simulink model "RemoteMicrogrid"  (R2025a)
settings: Solver=FixedStepAuto  StartTime=0.0  StopTime=8  FixedStep=Ts  MaxStep=1e-3  RelTol=1e-3
PreLoadFcn:
  | RemoteMicrogridInputData
undefined symbols (not defined in the file): BESS, ControlRoom, DiscIntNeverNeededParam, Grid, Load, Machine, Microgrid, MicrogridStatus, PV, relay1, T_on, Ts
libraries: ee_lib x53, fl_lib x39, eeGeneralControl x30, simulink x30, nesl_utility x26, nesl_utility_internal x19, slpidlib x7, eeTransforms x5, eeRmsMeasurement x4, eeTotalHarmonicDistorsion x4, batteryecm_lib x2, simulink_extras x2
(part 2 of 6)

== system RemoteMicrogrid/Diesel Substation, BESS, & Microgrid Controller/Diesel Generator ==
  Bus Element In : Inport  PortName=MGController  Element=Status.loadReference
  AVR and Exciter : Subsystem
  Add : Sum
  Constant : Constant  Value=Machine.LoadReference
  "Governor and Prime Mover " : Subsystem  mask(Governor and Prime Mover){pu_speed_reference=Machine.SpeedReference, droop_percentage=Machine.Droop, pu_load_reference_setpoint=Machine.LoadReference, T_G=Machine.TimeConstandGovernor, T_CH=Machine.TimeConstantPrimeMover, base_torque=Machine.BaseTorque, pu_torque0=Machine.InitialTorque}
      mask prompts: pu_speed_reference "Speed reference, (pu)"; droop_percentage "Percentage droop, (%)"; pu_load_reference_setpoint "Load reference setpoint, (pu)"; T_G "Time constant of governor, (s)"; T_CH "Time constant of main inlet volumes and steam chest, (s)"; base_torque "Base torque, (N*m)"; pu_torque0 "Initial torque, (pu)"
      mask help:
      | Implements a synchronous machine governor and prime mover. The prime mover is a non-reheat steam turbine.
      |
      | The input to the block is a per-unit synchronous machine measurement vector.
      |
      | R and C are mechanical rotational ports.
  Machine Inertia : ee_lib/Electromechanical/Mechanical/Machine Inertia  SRated=Grid.DieselRatedPower V*A  FRated=Grid.Frequency Hz  nPolePairs=1  inertia_option=1  J=Machine.Inertia kg*m^2  H=3.525 s*W/V/A  damper_option=2  D=39.0509 N*m/(rad/s)  pu_D=0.01  initialization_option=2  fMechanical0=60 Hz  fElectrical0=Grid.Frequency Hz
      settings: InternalSimscapePortConfiguration="{\"Bottom\":[],\"Left\":[{\"id\":\"R\",\"label\":\"R\",\"type\":\"foundation.mechanical.rotational.rotational\"}],\"Right\":[],\"Top\":[]}"
  Synchronous Machine Round Rotor : ee_lib/Electromechanical/Synchronous/Synchronous Machine Round Rotor  port_option=ee.enum.threePhasePort.composite  SRated=Grid.DieselRatedPower A*V  VRated=Grid.Voltage V  FRated=Grid.Frequency Hz  nPolePairs=1  param_option=ee.enum.sm.parameterization.standard  fieldCircuitParameterization_option=ee.enum.sm.fieldparameterization.current  baseEfd=92.95 V  baseIfd=1300 A  zero_sequence=ee.enum.park.zerosequence.include  axes_param=ee.enum.rotorangle.daxis  Ladu=1.66  Laqu=1.61  L0=0.15  Ll=0.05  Ra=0.03  Lfd=0.165  Rfd=0.0006  L1d=0.1713  R1d=0.0284  L1q=0.7252  R1q=0.00619  L2q=0.125  R2q=0.02368  Xl=0.05  Xd=1.72  Xq=0.79  X0=0.06  Xdd=0.13  Xqd=0.17  Xddd=0.09  Xqdd=0.12  d_option=ee.enum.circuit.open  Td0d=0.75 s  Tdd=0.03 s  Td0dd=0.03 s  Tddd=0.008 s  q_option=ee.enum.circuit.open  Tq0d=0.6 s  Tqd=0.03 s  Tq0dd=0.02 s  Tqdd=0.008 s  saturation_option=ee.enum.saturation.exclude  saturation_ifd=[0, .48, .76, 1.38, 1.79]  saturation_Vag=[0, .8, 1.08, 1.31, 1.4]  initialization_option=ee.enum.sm.initialization.steadystate  source_type=ee.enum.sm.load_flow_source_type.Swing  Vmag0=Grid.Voltage V  Vang0=0 deg  Pt0=Grid.DieselRatedPower A*V  Qt0=0 A*V  minimum_pu=0.95  phase_search_range=[-inf, inf] deg  gmin=1e-6 S  connection_option=ee.enum.Connection.wye  num_q_dampers=2  rotor_offset=-pi / 2 rad  pu_psid_specify=off  pu_psid_priority=None  pu_psid=0  pu_psid_nominal_specify=off  pu_psid_nominal_value=1  pu_psid_nominal_unit=1  pu_psiq_specify=off  pu_psiq_priority=None  pu_psiq=0  pu_psiq_nominal_specify=off  pu_psiq_nominal_value=1  pu_psiq_nominal_unit=1  pu_psifd_specify=off  pu_psifd_priority=None  pu_psifd=0  pu_psifd_nominal_specify=off  pu_psifd_nominal_value=1  pu_psifd_nominal_unit=1  pu_psi1d_specify=off  pu_psi1d_priority=None  pu_psi1d=0  pu_psi1d_nominal_specify=off  pu_psi1d_nominal_value=1  pu_psi1d_nominal_unit=1  pu_psi1q_specify=off  pu_psi1q_priority=None  pu_psi1q=0  pu_psi1q_nominal_specify=off  pu_psi1q_nominal_value=1  pu_psi1q_nominal_unit=1  pu_psi2q_specify=off  pu_psi2q_priority=None  pu_psi2q=0  pu_psi2q_nominal_specify=off  pu_psi2q_nominal_value=1  pu_psi2q_nominal_unit=1  angular_position_diff_specify=off  angular_position_diff_priority=None  angular_position_diff=180 deg  angular_position_diff_nominal_specify=off  angular_position_diff_nominal_value=1  angular_position_diff_nominal_unit=deg  Tmeas=298.15 K  alpha=3.93e-3 1/K  stator_thermal_mass=100 J/K  rotor_thermal_mass=200 J/K  temperatureA_specify=off  temperatureA_priority=High  temperatureA=25 degC  temperatureA_nominal_specify=off  temperatureA_nominal_value=1  temperatureA_nominal_unit=degC  temperatureB_specify=off  temperatureB_priority=High  temperatureB=25 degC  temperatureB_nominal_specify=off  temperatureB_nominal_value=1  temperatureB_nominal_unit=degC  temperatureC_specify=off  temperatureC_priority=High  temperatureC=25 degC  temperatureC_nominal_specify=off  temperatureC_nominal_value=1  temperatureC_nominal_unit=degC  temperatureR_specify=off  temperatureR_priority=High  temperatureR=25 degC  temperatureR_nominal_specify=off  temperatureR_nominal_value=1  temperatureR_nominal_unit=degC
      settings: InternalSimscapePortConfiguration="{\"Bottom\":[],\"Left\":[{\"id\":\"fd_p\",\"label\":\"fd+\",\"type\":\"foundation.electrical.electrical\"},{\"id\":\"fd_n\",\"label\":\"fd-\",\"type\":\"foundation.electrical.electrical\"},{\"id\":\"R\",\"label\":\"R\",\"type\":\"foundation.mechanical.rotational.rotational\"},{\"id\":\"C\",\"label\":\"C\",\"type\":\"foundation.mechanical.rotational.rotational\"}],\"Right\":[{\"id\":\"pu_output\",\"label\":\"pu\",\"type\":\"output\"},{\"id\":\"N\",\"label\":\"~\",\"type\":\"foundation.electrical.three_phase\"},{\"id\":\"n\",\"label\":\"n\",\"type\":\"foundation.electrical.electrical\"}],\"Top\":[]}"
  ref : PMIOPort  Side=Left
  ~ : PMIOPort  Port=2  Side=Right
  wires:
  Add/1 -> "Governor and Prime Mover "/1(Load)
  Constant/1 -> Add/2
  Bus Element In/1 -> Add/1
  connections:
  AVR and Exciter/LConn1 -- "Governor and Prime Mover "/LConn1 -- Synchronous Machine Round Rotor/RConn1
  Synchronous Machine Round Rotor/LConn3 -- Machine Inertia/LConn1 -- "Governor and Prime Mover "/RConn1
  Synchronous Machine Round Rotor/LConn1 -- AVR and Exciter/RConn1
  AVR and Exciter/RConn2 -- Synchronous Machine Round Rotor/RConn3 -- ref/RConn1 -- Synchronous Machine Round Rotor/LConn2
  Synchronous Machine Round Rotor/LConn4 -- "Governor and Prime Mover "/RConn2
  Synchronous Machine Round Rotor/RConn2 -- ~/RConn1

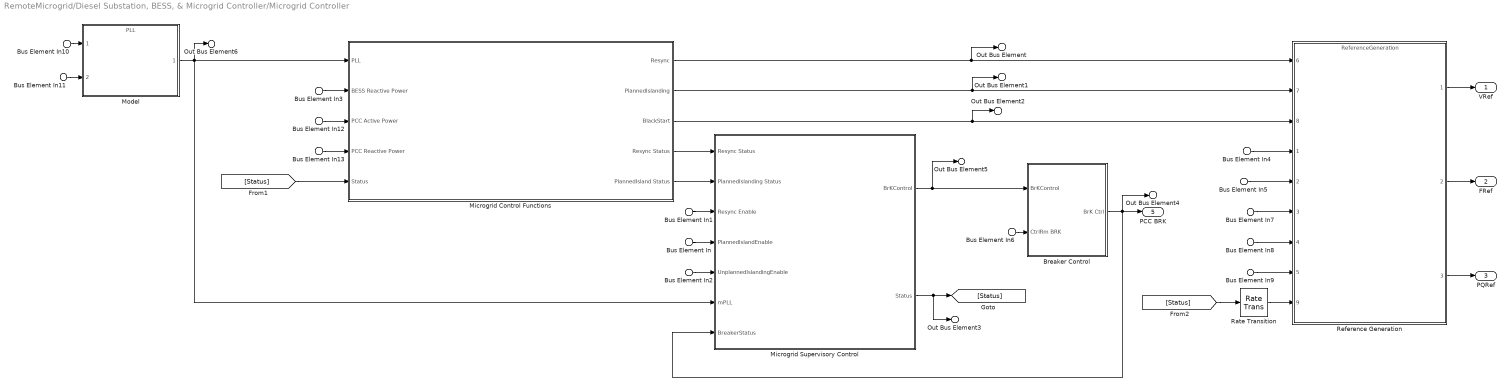
== system RemoteMicrogrid/Diesel Substation, BESS, & Microgrid Controller/Microgrid Controller ==
  Bus Element In3 : Inport  PortName=CtrlRmSubstation  Element=BESSReactivePower
  Bus Element In4 : Inport  PortName=CtrlRmSubstation  Element=Pref
  Bus Element In5 : Inport  PortName=CtrlRmSubstation  Element=Qref
  Bus Element In7 : Inport  PortName=CtrlRmSubstation  Element=Vref
  Bus Element In8 : Inport  PortName=CtrlRmSubstation  Element=Fref
  Bus Element In9 : Inport  PortName=CtrlRmSubstation  Element=PowerCmd
  Bus Element In : Inport  PortName=CtrlRmSubstation  Element=PlannedIslandCmd
  Bus Element In1 : Inport  PortName=CtrlRmSubstation  Element=ResynchCmd
  Bus Element In2 : Inport  PortName=CtrlRmSubstation  Element=UnplannedIslanding
  Bus Element In6 : Inport  PortName=CtrlRmSubstation  Element=BRKcontrol
  Bus Element In10 : Inport  Port=2  PortName=mPCC  Element=Grid.voltage
  Bus Element In11 : Inport  Port=2  PortName=mPCC  Element=PCC.voltage
  Bus Element In12 : Inport  Port=2  PortName=mPCC  Element=PCC.activePower
  Bus Element In13 : Inport  Port=2  PortName=mPCC  Element=PCC.reactivePower
  Breaker Control : Subsystem  mask(Breaker Control){}
      mask help: Control breaker at PCC
  Microgrid Control Functions : Subsystem
  Microgrid Supervisory Control : Subsystem
  Model : ModelReference  ModelNameDialog=PLL.slx  UsingDefaultArgumentValue=0,0,0  SimulationMode=Normal  ModelReferenceVersion=5.0  GridFrequency=gridFrequency  KiPLLController=kpPLL  KpPLLController=kiPLL
  Rate Transition : RateTransition  OutPortSampleTime=1e-3
  Reference Generation : ModelReference  ModelNameDialog=ReferenceGeneration.slx  UsingDefaultArgumentValue=0,0,0,0,0  SimulationMode=Normal  ModelReferenceVersion=5.0  GridFrequency=gridFrequency  pUpperLimit=pUpperLimit  pLowerLimit=pLowerLimit  qUpperLimit=qUpperLimit  qLowerLimit=qLowerLimit
      settings: PortSchema="{\"entries\":[{\"content\":{\"sides\":[{\"content\":{\"connectorIds\":[\"In6\",\"In7\",\"In8\",\"In1\",\"In2\",\"In3\",\"In4\",\"In5\",\"In9\"]},\"type\":\"ConnectorPlacement.EquallySpacedRectSide\",\"uuid\":\"e872b833-49f6-4912-b4b3-51343786db27\"},{\"content\":{\"connectorIds\":[\"Out1\",\"Out2\",\"Out3\"],\"side\":\"RIGHT\"},\"type\":\"ConnectorPlacement.EquallySpacedRectSide\",\"uuid\":\"d01ecec0-b655-4b5d-a34d-324f522879ad\"},{\"content\":{\"side\":\"TOP\"},\"type\":\"ConnectorPlacement.EquallySpacedRectSide\",\"uuid\":\"07b88f4e-1122-4691-94e1-fc20c2cbb47d\"}]},\"type\":\"ConnectorPlacement.EquallySpacedConnector\",\"uuid\":\"8d1da379-bdae-48c1-83d9-0dc3b93882b1\"}],\"packageUris\":[\"http://schema.mathworks.com/mf0/Connector/R2020b\"],\"version\":\"1.0\"}"
  VRef : Outport
  FRef : Outport  Port=2
  PQRef : Outport  Port=3
  Out Bus Element : Outport  Port=4  PortName=MGController  Element=Resync
  Out Bus Element1 : Outport  Port=4  PortName=MGController  Element=PlannedIslanding
  Out Bus Element2 : Outport  Port=4  PortName=MGController  Element=BlackStart
  Out Bus Element3 : Outport  Port=4  PortName=MGController  Element=Status
  Out Bus Element4 : Outport  Port=4  PortName=MGController  Element=BRK Status
  Out Bus Element6 : Outport  Port=4  PortName=MGController  Element=mPLL
  Out Bus Element5 : Outport  Port=4  PortName=MGController  Element=BrKControl
  PCC BRK : Outport  Port=5
  wires:
  Bus Element In7/1 -> Reference Generation/3
  Reference Generation/2 -> FRef/1
  Bus Element In8/1 -> Reference Generation/4
  Bus Element In3/1 -> Microgrid Control Functions/2(BESS Reactive Power)
  Reference Generation/1 -> VRef/1
  Reference Generation/3 -> PQRef/1
  Bus Element In12/1 -> Microgrid Control Functions/3(PCC Active Power)
  Bus Element In4/1 -> Reference Generation/1
  Bus Element In13/1 -> Microgrid Control Functions/4(PCC Reactive Power)
  Bus Element In10/1 -> Model/1
  Bus Element In5/1 -> Reference Generation/2
  Bus Element In2/1 -> Microgrid Supervisory Control/5(UnplannedIslandingEnable)
  Bus Element In/1 -> Microgrid Supervisory Control/4(PlannedIslandEnable)
  Bus Element In11/1 -> Model/2
  Bus Element In9/1 -> Reference Generation/5
  Bus Element In1/1 -> Microgrid Supervisory Control/3(Resync Enable)
  Microgrid Supervisory Control/1(BrKControl) -> Out Bus Element5/1, Breaker Control/1(BrKControl)
  Bus Element In6/1 -> Breaker Control/2(CtrlRm BRK)
  Model/1 -> Out Bus Element6/1, Microgrid Supervisory Control/6(mPLL), Microgrid Control Functions/1(PLL)
  Microgrid Control Functions/2(PlannedIslanding) -> Out Bus Element1/1, Reference Generation/7
  Microgrid Control Functions/1(Resync) -> Out Bus Element/1, Reference Generation/6
  Microgrid Control Functions/4(Resync Status) -> Microgrid Supervisory Control/1(Resync Status)
  Microgrid Control Functions/5(PlannedIsland Status) -> Microgrid Supervisory Control/2(PlannedIslanding Status)
  Breaker Control/1(BrK Ctrl) -> Microgrid Supervisory Control/7(BreakerStatus), PCC BRK/1, Out Bus Element4/1
  Microgrid Control Functions/3(BlackStart) -> Out Bus Element2/1, Reference Generation/8
  Microgrid Supervisory Control/2(Status) -> Out Bus Element3/1, [Status]
  [Status] -> Microgrid Control Functions/5(Status)
  [Status] -> Rate Transition/1
  Rate Transition/1 -> Reference Generation/9

== system RemoteMicrogrid/Diesel Substation, BESS, & Microgrid Controller/PCC Measurements and PCC Breaker ==
  Breaker : Inport
  Bus Creator : BusCreator  Inputs=2
  Circuit Breaker : Subsystem
  Diesel Genset Current Measurement : Subsystem
  Diesel Genset Power Measurement : Subsystem
  ~ : PMIOPort  Side=Left
  "~ " : PMIOPort  Port=2  Side=Right
  " mPCC" : Outport
  wires:
  Bus Creator/1 -> " mPCC"/1  "mPCC"
  Diesel Genset Power Measurement/1(PCC) -> Bus Creator/2  "PCC"
  Diesel Genset Current Measurement/1(Grid) -> Bus Creator/1  "Grid"
  Breaker/1 -> Circuit Breaker/1(BRK)
  connections:
  Circuit Breaker/LConn1 -- Diesel Genset Current Measurement/RConn1
  Diesel Genset Power Measurement/RConn1 -- "~ "/RConn1
  ~/RConn1 -- Diesel Genset Current Measurement/LConn1
  Circuit Breaker/RConn1 -- Diesel Genset Power Measurement/LConn1

== system RemoteMicrogrid/Diesel Substation, BESS, & Microgrid Controller/Transformer and Disconnectors ==
  Connectors : ee_lib/Passive/RLC Assemblies/RLC (Three-Phase)  port_option=ee.enum.threePhasePort.composite  component_structure=ee.enum.rlc.structure.R  R=Grid.ConnectorResistance Ohm  L=0.01 H  C=1e-6 F  R_parasitic=1e-6 Ohm  G_parasitic=1e-6 1/Ohm  IL_specify=on  IL_priority=High  IL=[0, 0, 0] A  IL_nominal_specify=off  IL_nominal_value=1  IL_nominal_unit=A  VC_specify=off  VC_priority=High  VC=[0, 0, 0] V  VC_nominal_specify=off  VC_nominal_value=1  VC_nominal_unit=V
      settings: InternalSimscapePortConfiguration="{\"Bottom\":[],\"Left\":[{\"id\":\"N1\",\"label\":\"~1\",\"type\":\"foundation.electrical.three_phase\"}],\"Right\":[{\"id\":\"N2\",\"label\":\"~2\",\"type\":\"foundation.electrical.three_phase\"}],\"Top\":[]}"
  Electrical Reference5 : fl_lib/Electrical/Electrical Elements/Electrical Reference
  Fault (Three-Phase) : ee_lib/Utilities/Fault (Three-Phase)  fault_type_option=1  R_pn_fault=50 Ohm  R_ng_fault=1e-3 Ohm  exposemeasurement=ee.enum.exposemeasurement.hidden  enable_external_fault=ee.enum.external_fault.hidden  fault_threshold=0.5  fault_condition=1  fault_resettable=1  enable_temporal_fault=1  fault_start_time=ControlRoom.unplannedIslanding s  fault_duration=0.3 s  G_parasitic=1e-6 1/Ohm
      settings: InternalSimscapePortConfiguration="{\"Bottom\":[],\"Left\":[{\"id\":\"N\",\"label\":\"~\",\"type\":\"foundation.electrical.three_phase\"}],\"Right\":[],\"Top\":[]}"
  Switchable 20 kW 4160 Vrms 60 Hz1 : ee_lib/Passive/RLC Assemblies/Wye-Connected Load  port_option=ee.enum.threePhasePort.composite  parameterization=ee.enum.rlc.parameterization.ratedpower  component_structure=ee.enum.rlc.structure.C  component_structure_PQ=ee.enum.rlc.structure.R  R=1 Ohm  L=0.001 H  C=1e-6 F  VRated=Microgrid.Voltage V  FRated=Grid.Frequency Hz  P=20000 W  Qpos=0 A*V  Qneg=-30000 A*V  R_parasitic=1e-6 Ohm  G_parasitic=1e-6 1/Ohm  R_parasitic_PQ=1e-6 Ohm  G_parasitic_PQ=1e-6 1/Ohm  Vmag0=Microgrid.Voltage V  Vang0=0 deg  Freq0=Microgrid.Frequency Hz  IL_specify=on  IL_priority=High  IL=[ 0 0 0 ] A  IL_nominal_specify=off  IL_nominal_value=1  IL_nominal_unit=A  VC_specify=on  VC_priority=High  VC=[ 0 0 0 ] V  VC_nominal_specify=off  VC_nominal_value=1  VC_nominal_unit=V
  Two-Winding Transformer (Three-Phase)1 : ee_lib/Passive/Transformers/Two-Winding Transformer (Three-Phase)  SRated=Grid.TransformerRating A*V  FRated=Grid.Frequency Hz  Winding1Connection=ee.enum.windingconnection.Y  VRated1=Grid.TransformerPrimaryVoltage V  Winding2Connection=ee.enum.windingconnection.Y  VRated2=Grid.TransformerSecondaryVoltage V  CoreType=ee.enum.coretype.threelimb  pu_Rw1=Grid.Primaryresistance  pu_Rw2=Grid.Secondaryresistance  leakage_reactance_option=ee.enum.transformer_leakage.include  pu_Xl1=Grid.Primaryreactance  pu_Xl2=Grid.Secondaryreactance  magnetizing_resistance_option=ee.enum.transformer_magnetizingResistance.include  pu_Rm=500  magnetizing_reactance_option=ee.enum.transformer_magnetizingReactance.include  saturation_option=ee.enum.transformer_saturation.exclude  pu_Xm=500  current_data=[0, .002, 1, 2]  magnetic_flux_data=[0, 1.2, 1.5, 1.51]  pu_X0=0.5  i1_specify=on  i1_priority=None  i1=[0, 0, 0] A  i1_nominal_specify=off  i1_nominal_value=1  i1_nominal_unit=A  i2_specify=on  i2_priority=None  i2=[0, 0, 0] A  i2_nominal_specify=off  i2_nominal_value=1  i2_nominal_unit=A  phi_specify=off  phi_priority=None  phi=[0, 0, 0]  phi_nominal_specify=off  phi_nominal_value=1  phi_nominal_unit=1  power_dissipated_specify=off  power_dissipated_priority=None  power_dissipated=0 W  power_dissipated_nominal_specify=off  power_dissipated_nominal_value=1  power_dissipated_nominal_unit=W
      settings: InternalSimscapePortConfiguration="{\"Bottom\":[],\"Left\":[{\"id\":\"N1\",\"label\":\"~1\",\"type\":\"foundation.electrical.three_phase\"}],\"Right\":[{\"id\":\"N2\",\"label\":\"~2\",\"type\":\"foundation.electrical.three_phase\"}],\"Top\":[]}"
  ~ : PMIOPort  Side=Left
  "~ " : PMIOPort  Port=2  Side=Right
  connections:
  Connectors/LConn1 -- Two-Winding Transformer (Three-Phase)1/RConn1
  Switchable 20 kW 4160 Vrms 60 Hz1/LConn1 -- "~ "/RConn1 -- Fault (Three-Phase)/LConn1 -- Connectors/RConn1
  Switchable 20 kW 4160 Vrms 60 Hz1/RConn1 -- Electrical Reference5/LConn1
  ~/RConn1 -- Two-Winding Transformer (Three-Phase)1/LConn1

== system RemoteMicrogrid/Feeder 2B & NO Switch/Circuit Breaker ==
  BRK : Inport
  Data Type Conversion : DataTypeConversion  OutDataTypeStr=double  SaturateOnIntegerOverflow=off  RndMeth=Floor
  Open Resistance : Gain  Gain=1e5
  Phase Splitter : ee_lib/Connectors & References/Phase Splitter
  Phase Splitter1 : ee_lib/Connectors & References/Phase Splitter
  Simulink-PS Converter : nesl_utility/Simulink-PS Converter  PhysicalDomain=network_engine_domain  SubClassName=ps_input  LeftPortType=input  RightPortType=output  PseudoPeriodic=off  Frequencies=[]  NoiseDistribution=none  NoiseParameters=[]  Unit=1  AffineConversion=off  FilteringAndDerivatives=provide  SimscapeFilterOrder=1  InputFilterTimeConstant=0.001  UdotUserProvided=0
  Variable Resistor : fl_lib/Electrical/Electrical Elements/Variable Resistor  Rmin=1e-3 Ohm  thermalEnable=false  thermal_mass=1 J/K  i_specify=off  i_priority=None  i=0 A  i_nominal_specify=off  i_nominal_value=1  i_nominal_unit=A  v_specify=off  v_priority=None  v=0 V  v_nominal_specify=off  v_nominal_value=1  v_nominal_unit=V  T_specify=off  T_priority=None  T=300 K  T_nominal_specify=off  T_nominal_value=1  T_nominal_unit=K
  Variable Resistor1 : fl_lib/Electrical/Electrical Elements/Variable Resistor  Rmin=1e-3 Ohm  thermalEnable=false  thermal_mass=1 J/K  i_specify=off  i_priority=None  i=0 A  i_nominal_specify=off  i_nominal_value=1  i_nominal_unit=A  v_specify=off  v_priority=None  v=0 V  v_nominal_specify=off  v_nominal_value=1  v_nominal_unit=V  T_specify=off  T_priority=None  T=300 K  T_nominal_specify=off  T_nominal_value=1  T_nominal_unit=K
  Variable Resistor2 : fl_lib/Electrical/Electrical Elements/Variable Resistor  Rmin=1e-3 Ohm  thermalEnable=false  thermal_mass=1 J/K  i_specify=off  i_priority=None  i=0 A  i_nominal_specify=off  i_nominal_value=1  i_nominal_unit=A  v_specify=off  v_priority=None  v=0 V  v_nominal_specify=off  v_nominal_value=1  v_nominal_unit=V  T_specify=off  T_priority=None  T=300 K  T_nominal_specify=off  T_nominal_value=1  T_nominal_unit=K
  In : PMIOPort  Side=Left
  ~ : PMIOPort  Port=2  Side=Right
  wires:
  Data Type Conversion/1 -> Open Resistance/1
  BRK/1 -> Data Type Conversion/1
  Open Resistance/1 -> Simulink-PS Converter/1
  connections:
  Phase Splitter1/RConn2 -- Variable Resistor1/RConn1
  Variable Resistor1/LConn2 -- Phase Splitter/RConn2
  Phase Splitter1/RConn3 -- Variable Resistor2/RConn1
  Phase Splitter/RConn1 -- Variable Resistor/LConn2
  Variable Resistor2/LConn2 -- Phase Splitter/RConn3
  Phase Splitter1/RConn1 -- Variable Resistor/RConn1
  Phase Splitter1/LConn1 -- ~/RConn1
  Variable Resistor/LConn1 -- Simulink-PS Converter/RConn1 -- Variable Resistor2/LConn1 -- Variable Resistor1/LConn1
  Phase Splitter/LConn1 -- In/RConn1

== system RemoteMicrogrid/Feeder 2B & NO Switch/Circuit Breaker1 ==
  BRK : Inport
  Data Type Conversion : DataTypeConversion  OutDataTypeStr=double  SaturateOnIntegerOverflow=off  RndMeth=Floor
  Open Resistance : Gain  Gain=1e5
  Phase Splitter : ee_lib/Connectors & References/Phase Splitter
  Phase Splitter1 : ee_lib/Connectors & References/Phase Splitter
  Simulink-PS Converter : nesl_utility/Simulink-PS Converter  PhysicalDomain=network_engine_domain  SubClassName=ps_input  LeftPortType=input  RightPortType=output  PseudoPeriodic=off  Frequencies=[]  NoiseDistribution=none  NoiseParameters=[]  Unit=1  AffineConversion=off  FilteringAndDerivatives=provide  SimscapeFilterOrder=1  InputFilterTimeConstant=0.001  UdotUserProvided=0
  Variable Resistor : fl_lib/Electrical/Electrical Elements/Variable Resistor  Rmin=1e-3 Ohm  thermalEnable=false  thermal_mass=1 J/K  i_specify=off  i_priority=None  i=0 A  i_nominal_specify=off  i_nominal_value=1  i_nominal_unit=A  v_specify=off  v_priority=None  v=0 V  v_nominal_specify=off  v_nominal_value=1  v_nominal_unit=V  T_specify=off  T_priority=None  T=300 K  T_nominal_specify=off  T_nominal_value=1  T_nominal_unit=K
  Variable Resistor1 : fl_lib/Electrical/Electrical Elements/Variable Resistor  Rmin=1e-3 Ohm  thermalEnable=false  thermal_mass=1 J/K  i_specify=off  i_priority=None  i=0 A  i_nominal_specify=off  i_nominal_value=1  i_nominal_unit=A  v_specify=off  v_priority=None  v=0 V  v_nominal_specify=off  v_nominal_value=1  v_nominal_unit=V  T_specify=off  T_priority=None  T=300 K  T_nominal_specify=off  T_nominal_value=1  T_nominal_unit=K
  Variable Resistor2 : fl_lib/Electrical/Electrical Elements/Variable Resistor  Rmin=1e-3 Ohm  thermalEnable=false  thermal_mass=1 J/K  i_specify=off  i_priority=None  i=0 A  i_nominal_specify=off  i_nominal_value=1  i_nominal_unit=A  v_specify=off  v_priority=None  v=0 V  v_nominal_specify=off  v_nominal_value=1  v_nominal_unit=V  T_specify=off  T_priority=None  T=300 K  T_nominal_specify=off  T_nominal_value=1  T_nominal_unit=K
  In : PMIOPort  Side=Left
  ~ : PMIOPort  Port=2  Side=Right
  wires:
  Data Type Conversion/1 -> Open Resistance/1
  BRK/1 -> Data Type Conversion/1
  Open Resistance/1 -> Simulink-PS Converter/1
  connections:
  Phase Splitter1/RConn2 -- Variable Resistor1/RConn1
  Variable Resistor1/LConn2 -- Phase Splitter/RConn2
  Phase Splitter1/RConn3 -- Variable Resistor2/RConn1
  Phase Splitter/RConn1 -- Variable Resistor/LConn2
  Variable Resistor2/LConn2 -- Phase Splitter/RConn3
  Phase Splitter1/RConn1 -- Variable Resistor/RConn1
  Phase Splitter1/LConn1 -- ~/RConn1
  Variable Resistor/LConn1 -- Simulink-PS Converter/RConn1 -- Variable Resistor2/LConn1 -- Variable Resistor1/LConn1
  Phase Splitter/LConn1 -- In/RConn1

== system RemoteMicrogrid/Feeder 2B & NO Switch/Subsystem ==
  ControlRoom : Inport
  Data Type Conversion1 : DataTypeConversion  SaturateOnIntegerOverflow=off  RndMeth=Floor
  Delay : Delay  DelayLength=6  SampleTime=0.15
  Logical Operator : Logic  Operator=NOT  AllPortsSameDT=off  OutDataTypeStr=boolean
  Output : Outport
  Output1 : Outport  Port=2
  wires:
  ControlRoom/1 -> Logical Operator/1, Delay/1
  Data Type Conversion1/1 -> Output1/1
  Delay/1 -> Data Type Conversion1/1
  Logical Operator/1 -> Output/1

== system RemoteMicrogrid/LV Load /Circuit Breaker ==
  BRK : Inport
  Data Type Conversion : DataTypeConversion  OutDataTypeStr=double  SaturateOnIntegerOverflow=off  RndMeth=Floor
  Gain : Gain  Gain=9.9e4
  Phase Splitter : ee_lib/Connectors & References/Phase Splitter
  Phase Splitter1 : ee_lib/Connectors & References/Phase Splitter
  Simulink-PS Converter : nesl_utility/Simulink-PS Converter  PhysicalDomain=network_engine_domain  SubClassName=ps_input  LeftPortType=input  RightPortType=output  PseudoPeriodic=off  Frequencies=[]  NoiseDistribution=none  NoiseParameters=[]  Unit=1  AffineConversion=off  FilteringAndDerivatives=provide  SimscapeFilterOrder=1  InputFilterTimeConstant=0.001  UdotUserProvided=0
  Variable Resistor : fl_lib/Electrical/Electrical Elements/Variable Resistor  Rmin=1e-3 Ohm  thermalEnable=false  thermal_mass=1 J/K  i_specify=off  i_priority=None  i=0 A  i_nominal_specify=off  i_nominal_value=1  i_nominal_unit=A  v_specify=off  v_priority=None  v=0 V  v_nominal_specify=off  v_nominal_value=1  v_nominal_unit=V  T_specify=off  T_priority=None  T=300 K  T_nominal_specify=off  T_nominal_value=1  T_nominal_unit=K
  Variable Resistor1 : fl_lib/Electrical/Electrical Elements/Variable Resistor  Rmin=1e-3 Ohm  thermalEnable=false  thermal_mass=1 J/K  i_specify=off  i_priority=None  i=0 A  i_nominal_specify=off  i_nominal_value=1  i_nominal_unit=A  v_specify=off  v_priority=None  v=0 V  v_nominal_specify=off  v_nominal_value=1  v_nominal_unit=V  T_specify=off  T_priority=None  T=300 K  T_nominal_specify=off  T_nominal_value=1  T_nominal_unit=K
  Variable Resistor2 : fl_lib/Electrical/Electrical Elements/Variable Resistor  Rmin=1e-3 Ohm  thermalEnable=false  thermal_mass=1 J/K  i_specify=off  i_priority=None  i=0 A  i_nominal_specify=off  i_nominal_value=1  i_nominal_unit=A  v_specify=off  v_priority=None  v=0 V  v_nominal_specify=off  v_nominal_value=1  v_nominal_unit=V  T_specify=off  T_priority=None  T=300 K  T_nominal_specify=off  T_nominal_value=1  T_nominal_unit=K
  In : PMIOPort  Side=Left
  ~ : PMIOPort  Port=2  Side=Right
  wires:
  Data Type Conversion/1 -> Gain/1
  BRK/1 -> Data Type Conversion/1
  Gain/1 -> Simulink-PS Converter/1
  connections:
  Phase Splitter1/RConn2 -- Variable Resistor1/RConn1
  Variable Resistor1/LConn2 -- Phase Splitter/RConn2
  Phase Splitter1/RConn3 -- Variable Resistor2/RConn1
  Phase Splitter/RConn1 -- Variable Resistor/LConn2
  Variable Resistor2/LConn2 -- Phase Splitter/RConn3
  Phase Splitter1/RConn1 -- Variable Resistor/RConn1
  Phase Splitter1/LConn1 -- ~/RConn1
  Variable Resistor/LConn1 -- Simulink-PS Converter/RConn1 -- Variable Resistor2/LConn1 -- Variable Resistor1/LConn1
  Phase Splitter/LConn1 -- In/RConn1

== system RemoteMicrogrid/LV Load /Circuit Breaker 1 ==
  BRK : Inport
  Data Type Conversion : DataTypeConversion  OutDataTypeStr=double  SaturateOnIntegerOverflow=off  RndMeth=Floor
  Gain : Gain  Gain=9.9e4
  Phase Splitter : ee_lib/Connectors & References/Phase Splitter
  Phase Splitter1 : ee_lib/Connectors & References/Phase Splitter
  Simulink-PS Converter : nesl_utility/Simulink-PS Converter  PhysicalDomain=network_engine_domain  SubClassName=ps_input  LeftPortType=input  RightPortType=output  PseudoPeriodic=off  Frequencies=[]  NoiseDistribution=none  NoiseParameters=[]  Unit=1  AffineConversion=off  FilteringAndDerivatives=provide  SimscapeFilterOrder=1  InputFilterTimeConstant=0.001  UdotUserProvided=0
  Variable Resistor : fl_lib/Electrical/Electrical Elements/Variable Resistor  Rmin=1e-3 Ohm  thermalEnable=false  thermal_mass=1 J/K  i_specify=off  i_priority=None  i=0 A  i_nominal_specify=off  i_nominal_value=1  i_nominal_unit=A  v_specify=off  v_priority=None  v=0 V  v_nominal_specify=off  v_nominal_value=1  v_nominal_unit=V  T_specify=off  T_priority=None  T=300 K  T_nominal_specify=off  T_nominal_value=1  T_nominal_unit=K
  Variable Resistor1 : fl_lib/Electrical/Electrical Elements/Variable Resistor  Rmin=1e-3 Ohm  thermalEnable=false  thermal_mass=1 J/K  i_specify=off  i_priority=None  i=0 A  i_nominal_specify=off  i_nominal_value=1  i_nominal_unit=A  v_specify=off  v_priority=None  v=0 V  v_nominal_specify=off  v_nominal_value=1  v_nominal_unit=V  T_specify=off  T_priority=None  T=300 K  T_nominal_specify=off  T_nominal_value=1  T_nominal_unit=K
  Variable Resistor2 : fl_lib/Electrical/Electrical Elements/Variable Resistor  Rmin=1e-3 Ohm  thermalEnable=false  thermal_mass=1 J/K  i_specify=off  i_priority=None  i=0 A  i_nominal_specify=off  i_nominal_value=1  i_nominal_unit=A  v_specify=off  v_priority=None  v=0 V  v_nominal_specify=off  v_nominal_value=1  v_nominal_unit=V  T_specify=off  T_priority=None  T=300 K  T_nominal_specify=off  T_nominal_value=1  T_nominal_unit=K
  In : PMIOPort  Side=Left
  ~ : PMIOPort  Port=2  Side=Right
  wires:
  Data Type Conversion/1 -> Gain/1
  BRK/1 -> Data Type Conversion/1
  Gain/1 -> Simulink-PS Converter/1
  connections:
  Phase Splitter1/RConn2 -- Variable Resistor1/RConn1
  Variable Resistor1/LConn2 -- Phase Splitter/RConn2
  Phase Splitter1/RConn3 -- Variable Resistor2/RConn1
  Phase Splitter/RConn1 -- Variable Resistor/LConn2
  Variable Resistor2/LConn2 -- Phase Splitter/RConn3
  Phase Splitter1/RConn1 -- Variable Resistor/RConn1
  Phase Splitter1/LConn1 -- ~/RConn1
  Variable Resistor/LConn1 -- Simulink-PS Converter/RConn1 -- Variable Resistor2/LConn1 -- Variable Resistor1/LConn1
  Phase Splitter/LConn1 -- In/RConn1

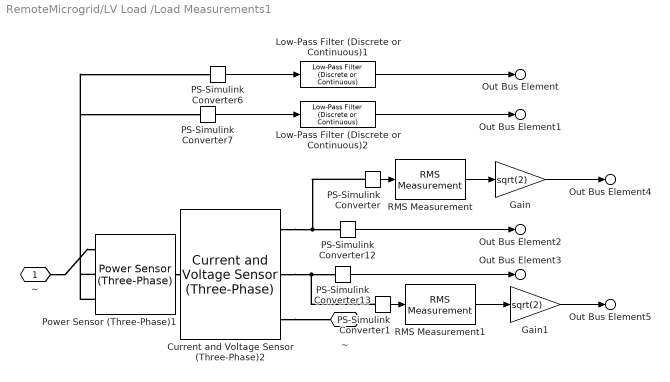
== system RemoteMicrogrid/LV Load /Load Measurements1 ==
  Current and Voltage Sensor (Three-Phase)2 : ee_lib/Sensors & Transducers/Current and Voltage Sensor (Three-Phase)  vMeasurementType=ee.enum.vmeasurement.ll  outputUnit=ee.enum.unit.pu  SRated=150e3 A*V  VRated=Microgrid.LVVoltage V  I_specify=off  I_priority=None  I=[0, 0, 0] A  I_nominal_specify=off  I_nominal_value=1  I_nominal_unit=A  V_specify=off  V_priority=None  V=[0, 0, 0] V  V_nominal_specify=off  V_nominal_value=1  V_nominal_unit=V
      settings: InternalSimscapePortConfiguration="{\"Bottom\":[],\"Left\":[{\"id\":\"N1\",\"label\":\"~1\",\"type\":\"foundation.electrical.three_phase\"}],\"Right\":[{\"id\":\"V_output\",\"label\":\"V\",\"type\":\"output\"},{\"id\":\"I_output\",\"label\":\"I\",\"type\":\"output\"},{\"id\":\"N2\",\"label\":\"~2\",\"type\":\"foundation.electrical.three_phase\"}],\"Top\":[]}"
  Gain : Gain  Gain=sqrt(2)
  Gain1 : Gain  Gain=sqrt(2)
  Low-Pass Filter (Discrete or Continuous)1 : eeGeneralControl/Low-Pass Filter (Discrete or Continuous)  K=1  T=0.02  B=inf  A=-inf  init_option=Inherited from block input  x0=0  Ts=Ts
  Low-Pass Filter (Discrete or Continuous)2 : eeGeneralControl/Low-Pass Filter (Discrete or Continuous)  K=1  T=0.02  B=inf  A=-inf  init_option=Inherited from block input  x0=0  Ts=Ts
  PS-Simulink Converter : nesl_utility/PS-Simulink Converter  PhysicalDomain=network_engine_domain  SubClassName=ps_output  LeftPortType=input  RightPortType=output  PseudoPeriodic=off  Frequencies=[]  VectorFormat=inherit  Unit=inherit  AffineConversion=off
  PS-Simulink Converter1 : nesl_utility/PS-Simulink Converter  PhysicalDomain=network_engine_domain  SubClassName=ps_output  LeftPortType=input  RightPortType=output  PseudoPeriodic=off  Frequencies=[]  VectorFormat=inherit  Unit=inherit  AffineConversion=off
  PS-Simulink Converter12 : nesl_utility_internal/PS-Simulink Converter  PhysicalDomain=network_engine_domain  SubClassName=ps_output  LeftPortType=input  RightPortType=output  PseudoPeriodic=off  Frequencies=[]  VectorFormat=1-D array  Unit=V  AffineConversion=off
  PS-Simulink Converter13 : nesl_utility_internal/PS-Simulink Converter  PhysicalDomain=network_engine_domain  SubClassName=ps_output  LeftPortType=input  RightPortType=output  PseudoPeriodic=off  Frequencies=[]  VectorFormat=1-D array  Unit=A  AffineConversion=off
  PS-Simulink Converter6 : nesl_utility_internal/PS-Simulink Converter  PhysicalDomain=network_engine_domain  SubClassName=ps_output  LeftPortType=input  RightPortType=output  PseudoPeriodic=off  Frequencies=[]  VectorFormat=1-D array  Unit=kW  AffineConversion=off
  PS-Simulink Converter7 : nesl_utility_internal/PS-Simulink Converter  PhysicalDomain=network_engine_domain  SubClassName=ps_output  LeftPortType=input  RightPortType=output  PseudoPeriodic=off  Frequencies=[]  VectorFormat=1-D array  Unit=kV*A  AffineConversion=off
  Power Sensor (Three-Phase)1 : ee_lib/Sensors & Transducers/Power Sensor (Three-Phase)  load_type=ee.enum.passive.type_balanced.balanced  f0=60 Hz  config=ee.enum.with_neutral.no  rho=1
      settings: InternalSimscapePortConfiguration="{\"Bottom\":[],\"Left\":[{\"id\":\"N1\",\"label\":\"~1\",\"type\":\"foundation.electrical.three_phase\"}],\"Right\":[{\"id\":\"N2\",\"label\":\"~2\",\"type\":\"foundation.electrical.three_phase\"}],\"Top\":[{\"id\":\"Pm\",\"label\":\"P\",\"type\":\"output\"},{\"id\":\"Qm\",\"label\":\"Q\",\"type\":\"output\"}]}"
  RMS Measurement : eeRmsMeasurement/RMS Measurement  LabelModeActiveChoice=Total  F=Grid.Frequency  SpecifyHarmonics=off  K=[0 1 2]  Ts=Ts
      settings: LibrarySourceBlock=|
      | ee_sl_lib/Measurements/RMS
      | Measurement
  RMS Measurement1 : eeRmsMeasurement/RMS Measurement  LabelModeActiveChoice=Total  F=Grid.Frequency  SpecifyHarmonics=off  K=[0 1 2]  Ts=Ts
      settings: LibrarySourceBlock=|
      | ee_sl_lib/Measurements/RMS
      | Measurement
  "~ " : PMIOPort  Side=Left
  " ~ " : PMIOPort  Port=2  Side=Right
  Out Bus Element : Outport  PortName=mLoadF2  Element=active powerF2
  Out Bus Element1 : Outport  PortName=mLoadF2  Element=reactive powerF2
  Out Bus Element2 : Outport  PortName=mLoadF2  Element=voltageF2
  Out Bus Element3 : Outport  PortName=mLoadF2  Element=currentF2
  Out Bus Element4 : Outport  PortName=mLoadF2  Element=voltageRMSF2
  Out Bus Element5 : Outport  PortName=mLoadF2  Element=currentRMSF2
  wires:
  Low-Pass Filter (Discrete or Continuous)2/1 -> Out Bus Element1/1
  Low-Pass Filter (Discrete or Continuous)1/1 -> Out Bus Element/1
  PS-Simulink Converter6/1 -> Low-Pass Filter (Discrete or Continuous)1/1
  PS-Simulink Converter7/1 -> Low-Pass Filter (Discrete or Continuous)2/1
  PS-Simulink Converter13/1 -> Out Bus Element3/1
  PS-Simulink Converter12/1 -> Out Bus Element2/1
  PS-Simulink Converter/1 -> RMS Measurement/1
  RMS Measurement/1 -> Gain/1
  RMS Measurement1/1 -> Gain1/1
  PS-Simulink Converter1/1 -> RMS Measurement1/1
  Gain/1 -> Out Bus Element4/1
  Gain1/1 -> Out Bus Element5/1
  connections:
  Power Sensor (Three-Phase)1/RConn1 -- Current and Voltage Sensor (Three-Phase)2/LConn1
  Current and Voltage Sensor (Three-Phase)2/RConn1 -- PS-Simulink Converter/LConn1 -- PS-Simulink Converter12/LConn1
  Current and Voltage Sensor (Three-Phase)2/RConn2 -- PS-Simulink Converter1/LConn1 -- PS-Simulink Converter13/LConn1
  "~ "/RConn1 -- Power Sensor (Three-Phase)1/LConn1
  Current and Voltage Sensor (Three-Phase)2/RConn3 -- " ~ "/RConn1
  Power Sensor (Three-Phase)1/LConn2 -- PS-Simulink Converter6/LConn1
  Power Sensor (Three-Phase)1/LConn3 -- PS-Simulink Converter7/LConn1

== system RemoteMicrogrid/MV Load/Circuit Breaker ==
  BRK : Inport
  Data Type Conversion : DataTypeConversion  OutDataTypeStr=double  SaturateOnIntegerOverflow=off  RndMeth=Floor
  Open Resistance : Gain  Gain=1e5
  Phase Splitter : ee_lib/Connectors & References/Phase Splitter
  Phase Splitter1 : ee_lib/Connectors & References/Phase Splitter
  Simulink-PS Converter : nesl_utility/Simulink-PS Converter  PhysicalDomain=network_engine_domain  SubClassName=ps_input  LeftPortType=input  RightPortType=output  PseudoPeriodic=off  Frequencies=[]  NoiseDistribution=none  NoiseParameters=[]  Unit=1  AffineConversion=off  FilteringAndDerivatives=provide  SimscapeFilterOrder=1  InputFilterTimeConstant=0.001  UdotUserProvided=0
  Variable Resistor : fl_lib/Electrical/Electrical Elements/Variable Resistor  Rmin=1e-3 Ohm  thermalEnable=false  thermal_mass=1 J/K  i_specify=off  i_priority=None  i=0 A  i_nominal_specify=off  i_nominal_value=1  i_nominal_unit=A  v_specify=off  v_priority=None  v=0 V  v_nominal_specify=off  v_nominal_value=1  v_nominal_unit=V  T_specify=off  T_priority=None  T=300 K  T_nominal_specify=off  T_nominal_value=1  T_nominal_unit=K
  Variable Resistor1 : fl_lib/Electrical/Electrical Elements/Variable Resistor  Rmin=1e-3 Ohm  thermalEnable=false  thermal_mass=1 J/K  i_specify=off  i_priority=None  i=0 A  i_nominal_specify=off  i_nominal_value=1  i_nominal_unit=A  v_specify=off  v_priority=None  v=0 V  v_nominal_specify=off  v_nominal_value=1  v_nominal_unit=V  T_specify=off  T_priority=None  T=300 K  T_nominal_specify=off  T_nominal_value=1  T_nominal_unit=K
  Variable Resistor2 : fl_lib/Electrical/Electrical Elements/Variable Resistor  Rmin=1e-3 Ohm  thermalEnable=false  thermal_mass=1 J/K  i_specify=off  i_priority=None  i=0 A  i_nominal_specify=off  i_nominal_value=1  i_nominal_unit=A  v_specify=off  v_priority=None  v=0 V  v_nominal_specify=off  v_nominal_value=1  v_nominal_unit=V  T_specify=off  T_priority=None  T=300 K  T_nominal_specify=off  T_nominal_value=1  T_nominal_unit=K
  In : PMIOPort  Side=Left
  ~ : PMIOPort  Port=2  Side=Right
  wires:
  Data Type Conversion/1 -> Open Resistance/1
  BRK/1 -> Data Type Conversion/1
  Open Resistance/1 -> Simulink-PS Converter/1
  connections:
  Phase Splitter1/RConn2 -- Variable Resistor1/RConn1
  Variable Resistor1/LConn2 -- Phase Splitter/RConn2
  Phase Splitter1/RConn3 -- Variable Resistor2/RConn1
  Phase Splitter/RConn1 -- Variable Resistor/LConn2
  Variable Resistor2/LConn2 -- Phase Splitter/RConn3
  Phase Splitter1/RConn1 -- Variable Resistor/RConn1
  Phase Splitter1/LConn1 -- ~/RConn1
  Variable Resistor/LConn1 -- Simulink-PS Converter/RConn1 -- Variable Resistor2/LConn1 -- Variable Resistor1/LConn1
  Phase Splitter/LConn1 -- In/RConn1

== system RemoteMicrogrid/MV Load/Circuit Breaker1 ==
  BRK : Inport
  Data Type Conversion : DataTypeConversion  OutDataTypeStr=double  SaturateOnIntegerOverflow=off  RndMeth=Floor
  Open Resistance : Gain  Gain=1e5
  Phase Splitter : ee_lib/Connectors & References/Phase Splitter
  Phase Splitter1 : ee_lib/Connectors & References/Phase Splitter
  Simulink-PS Converter : nesl_utility/Simulink-PS Converter  PhysicalDomain=network_engine_domain  SubClassName=ps_input  LeftPortType=input  RightPortType=output  PseudoPeriodic=off  Frequencies=[]  NoiseDistribution=none  NoiseParameters=[]  Unit=1  AffineConversion=off  FilteringAndDerivatives=provide  SimscapeFilterOrder=1  InputFilterTimeConstant=0.001  UdotUserProvided=0
  Variable Resistor : fl_lib/Electrical/Electrical Elements/Variable Resistor  Rmin=1e-3 Ohm  thermalEnable=false  thermal_mass=1 J/K  i_specify=off  i_priority=None  i=0 A  i_nominal_specify=off  i_nominal_value=1  i_nominal_unit=A  v_specify=off  v_priority=None  v=0 V  v_nominal_specify=off  v_nominal_value=1  v_nominal_unit=V  T_specify=off  T_priority=None  T=300 K  T_nominal_specify=off  T_nominal_value=1  T_nominal_unit=K
  Variable Resistor1 : fl_lib/Electrical/Electrical Elements/Variable Resistor  Rmin=1e-3 Ohm  thermalEnable=false  thermal_mass=1 J/K  i_specify=off  i_priority=None  i=0 A  i_nominal_specify=off  i_nominal_value=1  i_nominal_unit=A  v_specify=off  v_priority=None  v=0 V  v_nominal_specify=off  v_nominal_value=1  v_nominal_unit=V  T_specify=off  T_priority=None  T=300 K  T_nominal_specify=off  T_nominal_value=1  T_nominal_unit=K
  Variable Resistor2 : fl_lib/Electrical/Electrical Elements/Variable Resistor  Rmin=1e-3 Ohm  thermalEnable=false  thermal_mass=1 J/K  i_specify=off  i_priority=None  i=0 A  i_nominal_specify=off  i_nominal_value=1  i_nominal_unit=A  v_specify=off  v_priority=None  v=0 V  v_nominal_specify=off  v_nominal_value=1  v_nominal_unit=V  T_specify=off  T_priority=None  T=300 K  T_nominal_specify=off  T_nominal_value=1  T_nominal_unit=K
  In : PMIOPort  Side=Left
  ~ : PMIOPort  Port=2  Side=Right
  wires:
  Data Type Conversion/1 -> Open Resistance/1
  BRK/1 -> Data Type Conversion/1
  Open Resistance/1 -> Simulink-PS Converter/1
  connections:
  Phase Splitter1/RConn2 -- Variable Resistor1/RConn1
  Variable Resistor1/LConn2 -- Phase Splitter/RConn2
  Phase Splitter1/RConn3 -- Variable Resistor2/RConn1
  Phase Splitter/RConn1 -- Variable Resistor/LConn2
  Variable Resistor2/LConn2 -- Phase Splitter/RConn3
  Phase Splitter1/RConn1 -- Variable Resistor/RConn1
  Phase Splitter1/LConn1 -- ~/RConn1
  Variable Resistor/LConn1 -- Simulink-PS Converter/RConn1 -- Variable Resistor2/LConn1 -- Variable Resistor1/LConn1
  Phase Splitter/LConn1 -- In/RConn1

== system RemoteMicrogrid/MV Load/Load Measurements1 ==
  Current and Voltage Sensor (Three-Phase)2 : ee_lib/Sensors & Transducers/Current and Voltage Sensor (Three-Phase)  vMeasurementType=ee.enum.vmeasurement.ll  outputUnit=ee.enum.unit.pu  SRated=150e3 A*V  VRated=Microgrid.Voltage V  I_specify=off  I_priority=None  I=[0, 0, 0] A  I_nominal_specify=off  I_nominal_value=1  I_nominal_unit=A  V_specify=off  V_priority=None  V=[0, 0, 0] V  V_nominal_specify=off  V_nominal_value=1  V_nominal_unit=V
      settings: InternalSimscapePortConfiguration="{\"Bottom\":[],\"Left\":[{\"id\":\"N1\",\"label\":\"~1\",\"type\":\"foundation.electrical.three_phase\"}],\"Right\":[{\"id\":\"V_output\",\"label\":\"V\",\"type\":\"output\"},{\"id\":\"I_output\",\"label\":\"I\",\"type\":\"output\"},{\"id\":\"N2\",\"label\":\"~2\",\"type\":\"foundation.electrical.three_phase\"}],\"Top\":[]}"
  Gain : Gain  Gain=sqrt(2)
  Gain1 : Gain  Gain=sqrt(2)
  Low-Pass Filter (Discrete or Continuous)1 : eeGeneralControl/Low-Pass Filter (Discrete or Continuous)  K=1  T=0.02  B=inf  A=-inf  init_option=Inherited from block input  x0=0  Ts=Ts
  Low-Pass Filter (Discrete or Continuous)2 : eeGeneralControl/Low-Pass Filter (Discrete or Continuous)  K=1  T=0.02  B=inf  A=-inf  init_option=Inherited from block input  x0=0  Ts=Ts
  PS-Simulink Converter : nesl_utility/PS-Simulink Converter  PhysicalDomain=network_engine_domain  SubClassName=ps_output  LeftPortType=input  RightPortType=output  PseudoPeriodic=off  Frequencies=[]  VectorFormat=inherit  Unit=inherit  AffineConversion=off
  PS-Simulink Converter1 : nesl_utility_internal/PS-Simulink Converter  PhysicalDomain=network_engine_domain  SubClassName=ps_output  LeftPortType=input  RightPortType=output  PseudoPeriodic=off  Frequencies=[]  VectorFormat=1-D array  Unit=inherit  AffineConversion=off
  PS-Simulink Converter3 : nesl_utility/PS-Simulink Converter  PhysicalDomain=network_engine_domain  SubClassName=ps_output  LeftPortType=input  RightPortType=output  PseudoPeriodic=off  Frequencies=[]  VectorFormat=inherit  Unit=inherit  AffineConversion=off
  PS-Simulink Converter4 : nesl_utility_internal/PS-Simulink Converter  PhysicalDomain=network_engine_domain  SubClassName=ps_output  LeftPortType=input  RightPortType=output  PseudoPeriodic=off  Frequencies=[]  VectorFormat=1-D array  Unit=inherit  AffineConversion=off
  PS-Simulink Converter6 : nesl_utility_internal/PS-Simulink Converter  PhysicalDomain=network_engine_domain  SubClassName=ps_output  LeftPortType=input  RightPortType=output  PseudoPeriodic=off  Frequencies=[]  VectorFormat=1-D array  Unit=kW  AffineConversion=off
  PS-Simulink Converter7 : nesl_utility_internal/PS-Simulink Converter  PhysicalDomain=network_engine_domain  SubClassName=ps_output  LeftPortType=input  RightPortType=output  PseudoPeriodic=off  Frequencies=[]  VectorFormat=1-D array  Unit=kV*A  AffineConversion=off
  Power Sensor (Three-Phase)1 : ee_lib/Sensors & Transducers/Power Sensor (Three-Phase)  load_type=ee.enum.passive.type_balanced.balanced  f0=60 Hz  config=ee.enum.with_neutral.no  rho=1
      settings: InternalSimscapePortConfiguration="{\"Bottom\":[],\"Left\":[{\"id\":\"N1\",\"label\":\"~1\",\"type\":\"foundation.electrical.three_phase\"}],\"Right\":[{\"id\":\"N2\",\"label\":\"~2\",\"type\":\"foundation.electrical.three_phase\"}],\"Top\":[{\"id\":\"Pm\",\"label\":\"P\",\"type\":\"output\"},{\"id\":\"Qm\",\"label\":\"Q\",\"type\":\"output\"}]}"
  RMS Measurement : eeRmsMeasurement/RMS Measurement  LabelModeActiveChoice=Total  F=Grid.Frequency  SpecifyHarmonics=off  K=[0 1 2]  Ts=Ts
      settings: LibrarySourceBlock=|
      | ee_sl_lib/Measurements/RMS
      | Measurement
  RMS Measurement1 : eeRmsMeasurement/RMS Measurement  LabelModeActiveChoice=Total  F=Grid.Frequency  SpecifyHarmonics=off  K=[0 1 2]  Ts=Ts
      settings: LibrarySourceBlock=|
      | ee_sl_lib/Measurements/RMS
      | Measurement
  ~ : PMIOPort  Side=Left
  " ~ " : PMIOPort  Port=2  Side=Right
  Out Bus Element : Outport  PortName=mLoad  Element=active power
  Out Bus Element1 : Outport  PortName=mLoad  Element=reactive power
  Out Bus Element2 : Outport  PortName=mLoad  Element=voltage
  Out Bus Element3 : Outport  PortName=mLoad  Element=current
  Out Bus Element4 : Outport  PortName=mLoad  Element=voltageRMS
  Out Bus Element5 : Outport  PortName=mLoad  Element=currentRMS
  wires:
  PS-Simulink Converter7/1 -> Low-Pass Filter (Discrete or Continuous)2/1
  PS-Simulink Converter6/1 -> Low-Pass Filter (Discrete or Continuous)1/1
  Low-Pass Filter (Discrete or Continuous)1/1 -> Out Bus Element/1
  Low-Pass Filter (Discrete or Continuous)2/1 -> Out Bus Element1/1
  PS-Simulink Converter1/1 -> Out Bus Element2/1
  PS-Simulink Converter4/1 -> Out Bus Element3/1
  PS-Simulink Converter/1 -> RMS Measurement/1
  RMS Measurement/1 -> Gain1/1
  RMS Measurement1/1 -> Gain/1
  PS-Simulink Converter3/1 -> RMS Measurement1/1
  Gain/1 -> Out Bus Element4/1
  Gain1/1 -> Out Bus Element5/1
  connections:
  Power Sensor (Three-Phase)1/LConn3 -- PS-Simulink Converter7/LConn1
  Power Sensor (Three-Phase)1/LConn2 -- PS-Simulink Converter6/LConn1
  Current and Voltage Sensor (Three-Phase)2/RConn3 -- " ~ "/RConn1
  ~/RConn1 -- Power Sensor (Three-Phase)1/LConn1
  PS-Simulink Converter/LConn1 -- Current and Voltage Sensor (Three-Phase)2/RConn2 -- PS-Simulink Converter4/LConn1
  PS-Simulink Converter1/LConn1 -- PS-Simulink Converter3/LConn1 -- Current and Voltage Sensor (Three-Phase)2/RConn1
  Power Sensor (Three-Phase)1/RConn1 -- Current and Voltage Sensor (Three-Phase)2/LConn1

== system RemoteMicrogrid/Operator Control Room/Load Control ==
  Bus Element In : Inport  PortName=MGSubstation  Element=MGController.BrKControl.LoadF2A
  Bus Element In1 : Inport  PortName=MGSubstation  Element=MGController.BrKControl.LoadF2B
  Bus Element In2 : Inport  PortName=MGSubstation  Element=MGController.Status.loadDispatch
  Bus Element In3 : Inport  PortName=MGSubstation  Element=MGController.Status.loadDispatch
  Data Type Conversion{,1,3..4} (4 alike) : DataTypeConversion  OutDataTypeStr=double  SaturateOnIntegerOverflow=off  RndMeth=Floor
  Delay{,1..3} (4 alike) : Delay  DelayLength=1
  Step2 : Step  Time=Load.F1AControl  SampleTime=Ts
  Step3 : Step  Time=Load.F1BControl  SampleTime=Ts
  Step4 : Step  Time=Load.F2AControl  SampleTime=Ts
  Step6 : Step  Time=Load.F2AControl  SampleTime=Ts
  Switch : Switch  Criteria=u2 > Threshold  SaturateOnIntegerOverflow=off  InputSameDT=off
  Switch1 : Switch  Criteria=u2 > Threshold  SaturateOnIntegerOverflow=off  InputSameDT=off
  Out Bus Element12 : Outport  PortName=CtrlRmLoad  Element=Load1Control
  Out Bus Element4 : Outport  PortName=CtrlRmLoad  Element=Load2Control
  Out Bus Element5 : Outport  Port=2  PortName=CtrlRmF2Load  Element=Load2AControl
  Out Bus Element7 : Outport  Port=2  PortName=CtrlRmF2Load  Element=Load2BControl
  wires:
  Step2/1 -> Out Bus Element12/1
  Step3/1 -> Out Bus Element4/1
  Data Type Conversion3/1 -> Out Bus Element7/1
  Bus Element In/1 -> Delay/1
  Step6/1 -> Switch/3
  Switch/1 -> Data Type Conversion4/1
  Data Type Conversion4/1 -> Out Bus Element5/1
  Bus Element In1/1 -> Delay1/1
  Switch1/1 -> Data Type Conversion3/1
  Step4/1 -> Switch1/3
  Delay/1 -> Switch/1
  Bus Element In2/1 -> Data Type Conversion/1
  Delay1/1 -> Switch1/1
  Bus Element In3/1 -> Data Type Conversion1/1
  Delay2/1 -> Switch/2
  Delay3/1 -> Switch1/2
  Data Type Conversion/1 -> Delay2/1
  Data Type Conversion1/1 -> Delay3/1
